simulink model "control"  (R2017b)
settings: Solver=VariableStepAuto  StartTime=0.0  StopTime=2  RelTol=1e-3
values from neighbouring files (symbols this model uses):
  duracion = 1    [Controladores.m]
  n = 5    [Controladores.m]
  t_ini = 0.5    [Controladores.m]
  XYZfin = CinematicaDirecta([pi 3*pi/4 -pi/5])    [Controladores.m]
  XYZini = CinematicaDirecta([0 0 0])    [Controladores.m]
settings Model: Creator=fevaf  LastModifiedBy=fevaf

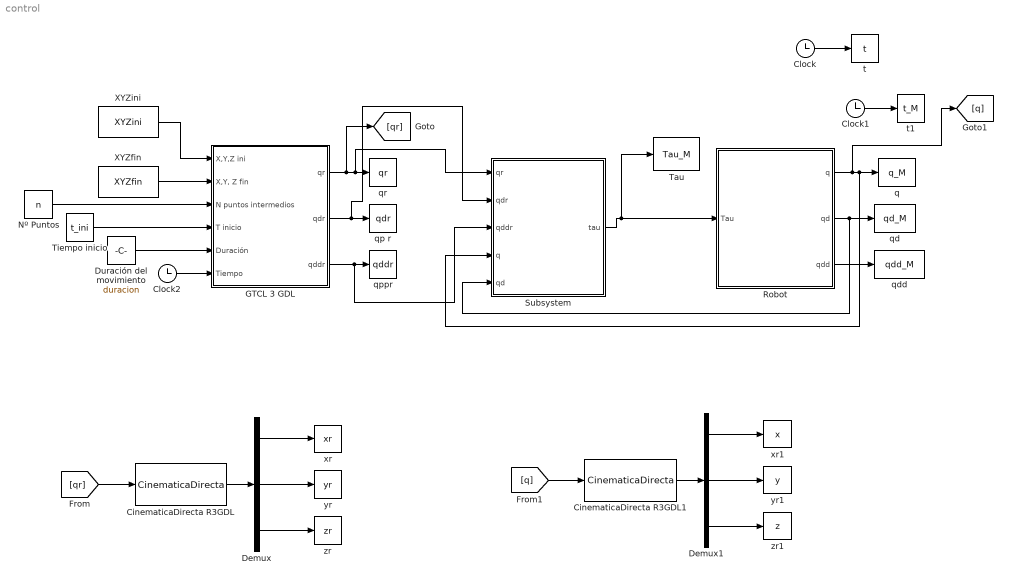
== system control ==
  CinematicaDirecta R3GDL : MATLABFcn  MATLABFcn=CinematicaDirecta
  CinematicaDirecta R3GDL1 : MATLABFcn  MATLABFcn=CinematicaDirecta
  Clock : Clock
  Clock1 : Clock
  Clock2 : Clock
  Demux : Demux  Outputs=3
  Demux1 : Demux  Outputs=3
  Duración del movimiento : Constant  Value=duracion
  GTCL 3 GDL : Subsystem
  Nº Puntos : Constant  Value=n
  Robot : Subsystem
  Subsystem : Subsystem
  "Tau " : ToWorkspace  VariableName=Tau_M  SampleTime=-1
  Tiempo inicio : Constant  Value=t_ini
  XYZfin : Constant  Value=XYZfin
  XYZini : Constant  Value=XYZini
  q : ToWorkspace  VariableName=q_M  SampleTime=-1
  qd : ToWorkspace  VariableName=qd_M  SampleTime=-1
  qdd : ToWorkspace  VariableName=qdd_M  SampleTime=-1
  qp r : ToWorkspace  VariableName=qdr  SampleTime=-1
  qppr : ToWorkspace  VariableName=qddr  SampleTime=-1
  qr : ToWorkspace  VariableName=qr  SampleTime=-1
  t : ToWorkspace  VariableName=t  SampleTime=-1
  t1 : ToWorkspace  VariableName=t_M  SampleTime=-1
  xr : ToWorkspace  VariableName=xr  SampleTime=-1
  xr1 : ToWorkspace  VariableName=x  SampleTime=-1
  yr : ToWorkspace  VariableName=yr  SampleTime=-1
  yr1 : ToWorkspace  VariableName=y  SampleTime=-1
  zr : ToWorkspace  VariableName=zr  SampleTime=-1
  zr1 : ToWorkspace  VariableName=z  SampleTime=-1
  wires:
  Demux/3 -> zr/1
  Demux/1 -> xr/1
  Demux/2 -> yr/1
  XYZfin/1 -> GTCL 3 GDL/2("X,Y, Z fin")
  XYZini/1 -> GTCL 3 GDL/1(X,Y,Z ini)
  Tiempo inicio/1 -> GTCL 3 GDL/4(T inicio)
  GTCL 3 GDL/3(qddr) -> Subsystem/3(qddr), qppr/1
  CinematicaDirecta R3GDL/1 -> Demux/1
  GTCL 3 GDL/1(qr) -> Subsystem/1(qr), qr/1, [qr]
  Clock2/1 -> GTCL 3 GDL/6(Tiempo)
  Duración del movimiento/1 -> GTCL 3 GDL/5(Duración)
  [qr] -> CinematicaDirecta R3GDL/1
  GTCL 3 GDL/2(qdr) -> Subsystem/2(qdr), qp r/1
  Nº Puntos/1 -> GTCL 3 GDL/3(N puntos intermedios)
  Clock/1 -> t/1
  Subsystem/1("tau ") -> Robot/1(Tau), "Tau "/1
  Robot/2(qd) -> Subsystem/5(qd), qd/1
  Robot/1(q) -> [q], Subsystem/4(q), q/1
  Robot/3(qdd) -> qdd/1
  Clock1/1 -> t1/1
  [q] -> CinematicaDirecta R3GDL1/1
  Demux1/2 -> yr1/1
  CinematicaDirecta R3GDL1/1 -> Demux1/1
  Demux1/3 -> zr1/1
  Demux1/1 -> xr1/1

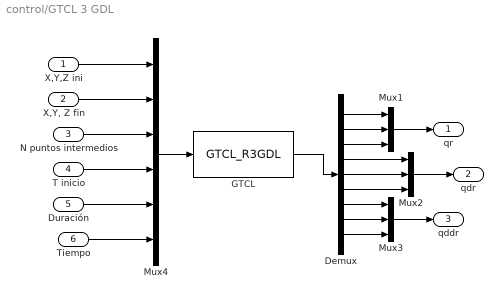
== system control/GTCL 3 GDL ==
  X,Y,Z ini : Inport
  "X,Y, Z fin" : Inport  Port=2
  N puntos intermedios : Inport  Port=3
  T inicio : Inport  Port=4
  Duración : Inport  Port=5
  Tiempo : Inport  Port=6
  Demux : Demux  Outputs=9
  GTCL : MATLABFcn  MATLABFcn=GTCL_R3GDL  OutputDimensions=9
  Mux1 : Mux  Inputs=3
  Mux2 : Mux  Inputs=3
  Mux3 : Mux  Inputs=3
  Mux4 : Mux  Inputs=6
  qr : Outport
  qdr : Outport  Port=2
  qddr : Outport  Port=3
  wires:
  Mux1/1 -> qr/1
  Mux4/1 -> GTCL/1
  X,Y,Z ini/1 -> Mux4/1
  "X,Y, Z fin"/1 -> Mux4/2
  N puntos intermedios/1 -> Mux4/3
  T inicio/1 -> Mux4/4
  Duración/1 -> Mux4/5
  Tiempo/1 -> Mux4/6
  GTCL/1 -> Demux/1
  Demux/1 -> Mux1/1
  Demux/2 -> Mux1/2
  Demux/3 -> Mux1/3
  Mux2/1 -> qdr/1
  Demux/4 -> Mux2/1
  Demux/5 -> Mux2/2
  Demux/6 -> Mux2/3
  Mux3/1 -> qddr/1
  Demux/7 -> Mux3/1
  Demux/8 -> Mux3/2
  Demux/9 -> Mux3/3

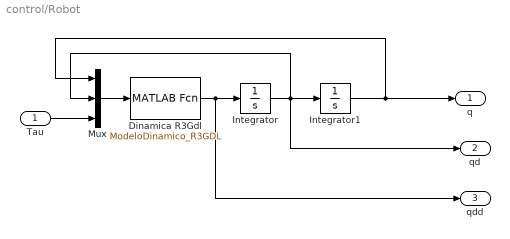
== system control/Robot ==
  Tau : Inport
  Dinamica R3Gdl : MATLABFcn  MATLABFcn=ModeloDinamico_R3GDL
  Integrator : Integrator  InitialCondition=[0;0;0];
  Integrator1 : Integrator  InitialCondition=[0;0;0]
  Mux : Mux  Inputs=3
  q : Outport
  qd : Outport  Port=2
  qdd : Outport  Port=3
  wires:
  Mux/1 -> Dinamica R3Gdl/1
  Dinamica R3Gdl/1 -> Integrator/1, qdd/1
  Integrator/1 -> Integrator1/1, qd/1, Mux/2
  Integrator1/1 -> q/1, Mux/1
  Tau/1 -> Mux/3

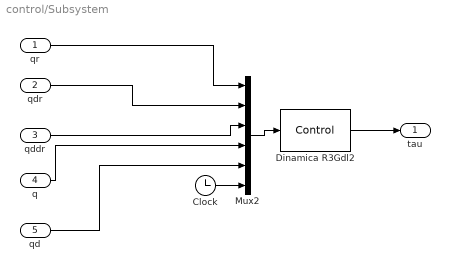
== system control/Subsystem ==
  qr : Inport
  qdr : Inport  Port=2
  qddr : Inport  Port=3
  q : Inport  Port=4
  qd : Inport  Port=5
  Clock : Clock
  Dinamica R3Gdl2 : MATLABFcn  MATLABFcn=Control  SampleTime=0.001
  Mux2 : Mux  Inputs=6
  "tau " : Outport
  wires:
  Mux2/1 -> Dinamica R3Gdl2/1
  Dinamica R3Gdl2/1 -> "tau "/1
  qr/1 -> Mux2/1
  qdr/1 -> Mux2/2
  qddr/1 -> Mux2/3
  q/1 -> Mux2/4
  qd/1 -> Mux2/5
  Clock/1 -> Mux2/6
